simulink model "Example1"  (R2022a)
settings: Solver=VariableStepAuto  StartTime=0.0  StopTime=20  RelTol=1e-3
undefined symbols (not defined in the file): K0, K1, K2, Ke0, Ke1
libraries: simulink x6
settings Model: Creator=mudit  LastModifiedBy=mudit

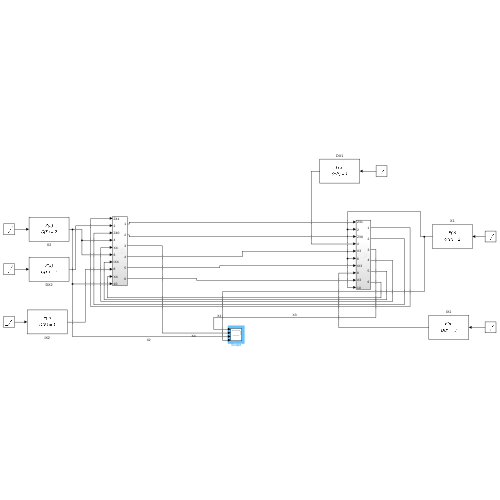
[thumbnail: Simulink's stored preview of the top-level diagram]
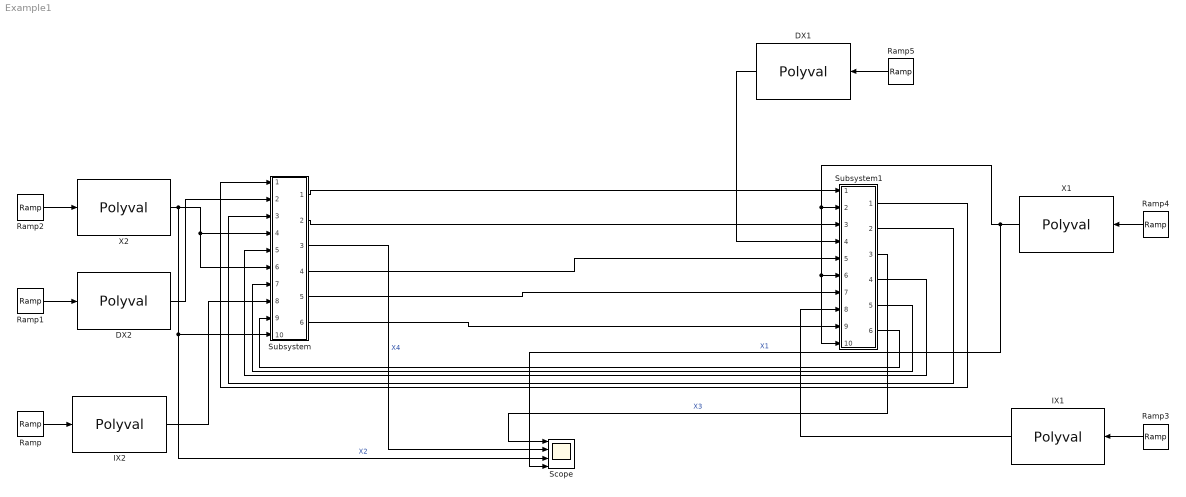
== system Example1 ==
  DX1 : Polyval  Coefs=[6,2]
  DX2 : Polyval  Coefs=[2,3]
  IX1 : Polyval  Coefs=[1,1,1,0]
  IX2 : Polyval  Coefs=[1/3,1.5,2,0]
  Ramp{,1..5} (6 alike) : simulink/Sources/Ramp  slope=1  start=0  InitialOutput=0
  Scope : Scope  NumInputPorts=4
  Subsystem : Subsystem
  Subsystem1 : Subsystem
  X1 : Polyval  Coefs=[3,2,1]
  X2 : Polyval  Coefs=[1,3,2]
  wires:
  Subsystem/1(Out2) -> Subsystem1/1(In1)
  Subsystem/4(Out1) -> Subsystem1/5(In5)
  Subsystem/5(Out3) -> Subsystem1/7(In7)
  Subsystem/6(Out4) -> Subsystem1/9(In9)
  Subsystem/2(Out5) -> Subsystem1/3(In3)
  Subsystem1/1(Out1) -> Subsystem/1(In1)
  Subsystem1/2(Out2) -> Subsystem/3(In3)
  Subsystem1/4(Out3) -> Subsystem/5(In5)
  Subsystem1/5(Out4) -> Subsystem/7(In7)
  Subsystem1/6(Out5) -> Subsystem/9(In9)
  X2/1 -> Scope/3, Subsystem/10(In10), Subsystem/6(In6), Subsystem/4(In4)  "X2"
  DX2/1 -> Subsystem/2(In2)
  X1/1 -> Scope/4, Subsystem1/10(In10), Subsystem1/6(In6), Subsystem1/2(In2)  "X1"
  DX1/1 -> Subsystem1/4(In4)
  IX1/1 -> Subsystem1/8(In8)
  IX2/1 -> Subsystem/8(In8)
  Ramp/1 -> IX2/1
  Ramp1/1 -> DX2/1
  Ramp2/1 -> X2/1
  Ramp5/1 -> DX1/1
  Ramp4/1 -> X1/1
  Ramp3/1 -> IX1/1
  Subsystem1/3(Out6) -> Scope/1  "X3"
  Subsystem/3(Out6) -> Scope/2  "X4"

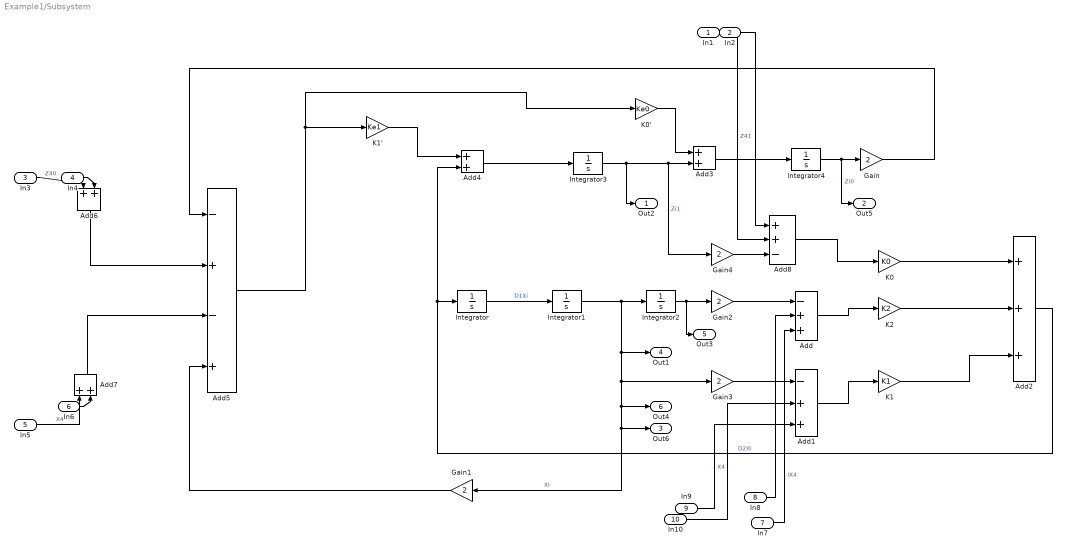
== system Example1/Subsystem ==
  In1 : Inport
  In2 : Inport  Port=2
  In3 : Inport  Port=3
  In4 : Inport  Port=4
  In5 : Inport  Port=5
  In6 : Inport  Port=6
  In7 : Inport  Port=7
  In8 : Inport  Port=8
  In9 : Inport  Port=9
  In10 : Inport  Port=10
  Add : Sum  Inputs=-++
  Add1 : Sum  Inputs=-++
  Add2 : Sum  Inputs=+++
  Add{3..4,6..7} (4 alike) : Sum
  Add5 : Sum  Inputs=-+-+
  Add8 : Sum  Inputs=++-
  Gain{,1..4} (5 alike) : Gain  Gain=2
  Integrator{,1..4} (5 alike) : Integrator
  K0 : Gain  Gain=K0
  K0' : Gain  Gain=Ke0
  K1 : Gain  Gain=K1
  K1' : Gain  Gain=Ke1
  K2 : Gain  Gain=K2
  Out2 : Outport
  Out5 : Outport  Port=2
  Out6 : Outport  Port=3
  Out1 : Outport  Port=4
  Out3 : Outport  Port=5
  Out4 : Outport  Port=6
  wires:
  Add1/1 -> K1/1
  Integrator3/1 -> Out2/1, Gain4/1, Add3/2  "Zi1"
  In8/1 -> Add/2
  K1'/1 -> Add4/1
  Gain2/1 -> Add/1
  In3/1 -> Add6/1  "Z40"
  K0'/1 -> Add3/1
  In5/1 -> Add7/1  "X4"
  Integrator4/1 -> Out5/1, Gain/1  "Zi0"
  Add7/1 -> Add5/3
  In6/1 -> Add7/2
  Add8/1 -> K0/1
  Integrator/1 -> Integrator1/1  "D1Xi"
  In1/1 -> Add8/2  "Z41"
  Add5/1 -> K0'/1, K1'/1
  Add4/1 -> Integrator3/1
  In4/1 -> Add6/2
  Add2/1 -> Add4/2, Integrator/1  "D2Xi"
  In10/1 -> Add1/2
  Gain1/1 -> Add5/4
  K2/1 -> Add2/2
  In7/1 -> Add/3  "IX4"
  In2/1 -> Add8/1
  Gain4/1 -> Add8/3
  Integrator1/1 -> Out1/1, Out4/1, Out6/1, Gain1/1, Gain3/1, Integrator2/1  "XI"
  In9/1 -> Add1/3  "X4"
  Gain3/1 -> Add1/1
  Add3/1 -> Integrator4/1
  Add6/1 -> Add5/2
  K0/1 -> Add2/1
  K1/1 -> Add2/3
  Integrator2/1 -> Out3/1, Gain2/1
  Add/1 -> K2/1
  Gain/1 -> Add5/1

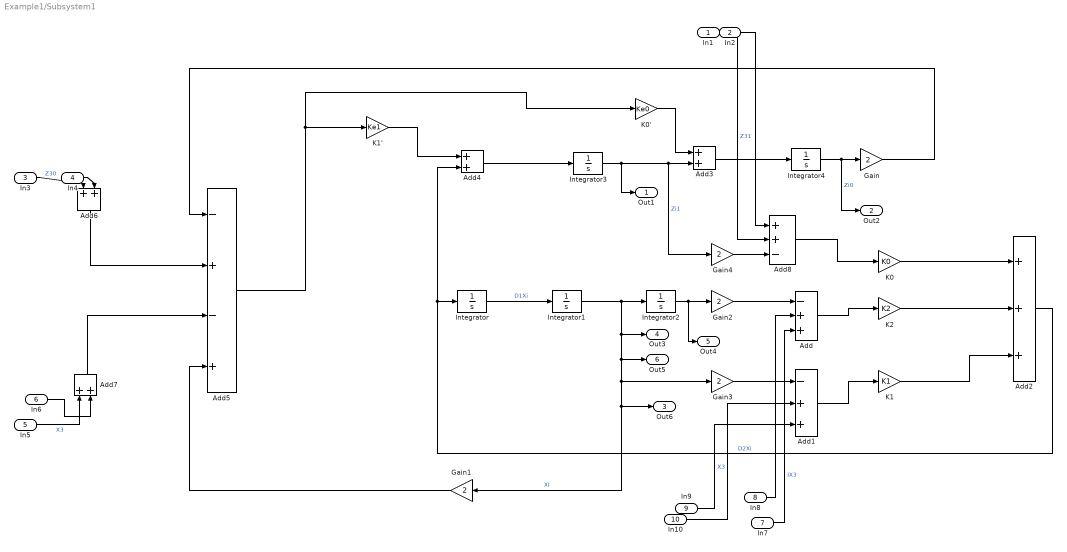
== system Example1/Subsystem1 ==
  In1 : Inport
  In2 : Inport  Port=2
  In3 : Inport  Port=3
  In4 : Inport  Port=4
  In5 : Inport  Port=5
  In6 : Inport  Port=6
  In7 : Inport  Port=7
  In8 : Inport  Port=8
  In9 : Inport  Port=9
  In10 : Inport  Port=10
  Add : Sum  Inputs=-++
  Add1 : Sum  Inputs=-++
  Add2 : Sum  Inputs=+++
  Add{3..4,6..7} (4 alike) : Sum
  Add5 : Sum  Inputs=-+-+
  Add8 : Sum  Inputs=++-
  Gain{,1..4} (5 alike) : Gain  Gain=2
  Integrator{,1..4} (5 alike) : Integrator
  K0 : Gain  Gain=K0
  K0' : Gain  Gain=Ke0
  K1 : Gain  Gain=K1
  K1' : Gain  Gain=Ke1
  K2 : Gain  Gain=K2
  Out1 : Outport
  Out2 : Outport  Port=2
  Out6 : Outport  Port=3
  Out3 : Outport  Port=4
  Out4 : Outport  Port=5
  Out5 : Outport  Port=6
  wires:
  Add1/1 -> K1/1
  Integrator3/1 -> Out1/1, Gain4/1, Add3/2  "Zi1"
  In8/1 -> Add/2
  K1'/1 -> Add4/1
  Gain2/1 -> Add/1
  In3/1 -> Add6/1  "Z30"
  K0'/1 -> Add3/1
  In5/1 -> Add7/1  "X3"
  Integrator4/1 -> Out2/1, Gain/1  "Zi0"
  Add7/1 -> Add5/3
  In6/1 -> Add7/2
  Add8/1 -> K0/1
  Integrator/1 -> Integrator1/1  "D1Xi"
  In1/1 -> Add8/2  "Z31"
  Add5/1 -> K0'/1, K1'/1
  Add4/1 -> Integrator3/1
  In4/1 -> Add6/2
  Add2/1 -> Add4/2, Integrator/1  "D2Xi"
  In10/1 -> Add1/2
  Gain1/1 -> Add5/4
  K2/1 -> Add2/2
  In7/1 -> Add/3  "IX3"
  In2/1 -> Add8/1
  Gain4/1 -> Add8/3
  Integrator1/1 -> Out3/1, Out6/1, Gain1/1, Gain3/1, Out5/1, Integrator2/1  "XI"
  In9/1 -> Add1/3  "X3"
  Gain3/1 -> Add1/1
  Add3/1 -> Integrator4/1
  Add6/1 -> Add5/2
  K0/1 -> Add2/1
  K1/1 -> Add2/3
  Integrator2/1 -> Out4/1, Gain2/1
  Add/1 -> K2/1
  Gain/1 -> Add5/1
